simulink model "dron_filtro_complementario_version2015_RP"  (R2015b)
settings: Solver=FixedStepDiscrete  StartTime=0.0  StopTime=inf  FixedStep=0.03  RelTol=1e-3
undefined symbols (not defined in the file): DiscIntNeverNeededParam
libraries: simulink x4, arduinolib x4, RASPlib x2
settings Model: SimulationMode=external  ExtModeTrigDuration=2  Creator=jorge  LastModifiedBy=jorge
settings OptimizationCC: OptimizeModelRefInitCode=on  LifeSpan=Inf  MaxStackSize=64
settings HardwareCC: ProdBitPerInt=16  ProdBitPerPointer=16  ProdLargestAtomicFloat=None  ProdWordSize=8  ProdHWDeviceType=Atmel->AVR
settings RTWCC: SystemTargetFile=ert.tlc  TemplateMakefile=ert_default_tmf  Description=Embedded Coder  Toolchain=Arduino AVR v1.6.1  BuildConfiguration=Faster Runs
settings CodeAppCC: IgnoreCustomStorageClasses=off
settings ERTTargetCC: SupportContinuousTime=on  SupportVariableSizeSignals=on  ExtMode=on  ExtModeMexFile=ext_serial_win32_comm_rtt  ExtModeMexArgs=0 5 115200

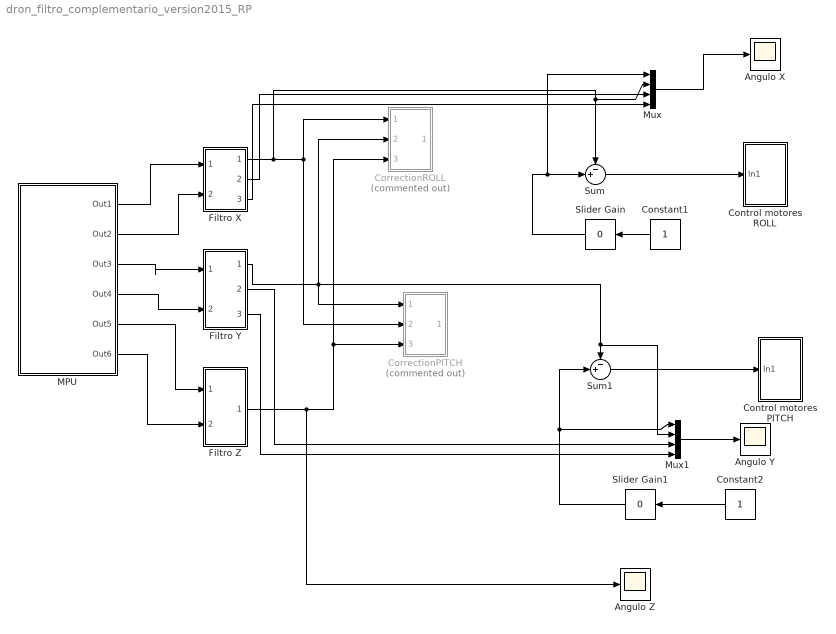
== system dron_filtro_complementario_version2015_RP ==
  Angulo X : Scope
  Angulo Y : Scope
  "Angulo Z " : Scope
  Constant1 : Constant
  Constant2 : Constant
  Control motores PITCH : Subsystem
  Control motores ROLL : Subsystem
  CorrectionPITCH : Subsystem  Commented=on
  CorrectionROLL : Subsystem  Commented=on
  Filtro X : Subsystem
  Filtro Y : Subsystem
  "Filtro Z " : Subsystem
  "MPU " : Subsystem
  Mux : Mux
  Mux1 : Mux
  Slider Gain : simulink/Math Operations/Slider Gain  low=-25  gain=0  high=35
  Slider Gain1 : simulink/Math Operations/Slider Gain  low=-25  gain=0  high=35
  Sum : Sum  Inputs=-+|
  Sum1 : Sum  Inputs=-+|
  wires:
  "MPU "/1(Out1) -> Filtro X/1(In1)
  "MPU "/2(Out2) -> Filtro X/2(In2)
  Mux/1 -> Angulo X/1
  Constant1/1 -> Slider Gain/1
  Slider Gain/1 -> Mux/1, Sum/2
  "MPU "/3(Out3) -> Filtro Y/1(In1)
  "MPU "/4(Out4) -> Filtro Y/2(In2)
  Sum/1 -> Control motores ROLL/1(In1)
  Constant2/1 -> Slider Gain1/1
  Sum1/1 -> Control motores PITCH/1(In1)
  Mux1/1 -> Angulo Y/1
  "MPU "/5(Out5) -> "Filtro Z "/1(In1)
  "MPU "/6(Out6) -> "Filtro Z "/2(In2)
  Filtro X/1(Out3) -> CorrectionPITCH/2(In2), CorrectionROLL/1(In1), Sum/1, Mux/2
  Filtro Y/1(Out3) -> CorrectionROLL/2(In2), Mux1/2, Sum1/1, CorrectionPITCH/1(In1)
  Slider Gain1/1 -> Mux1/1, Sum1/2
  "Filtro Z "/1(Out3) -> "Angulo Z "/1, CorrectionPITCH/3(In3), CorrectionROLL/3(In3)
  Filtro Y/2(Out1) -> Mux1/3
  Filtro Y/3(Out2) -> Mux1/4
  Filtro X/2(Out1) -> Mux/3
  Filtro X/3(Out2) -> Mux/4

== system dron_filtro_complementario_version2015_RP/Control motores PITCH ==
  In1 : Inport
  Control : Subsystem
  Motor1 : Subsystem
  Motor2 : Subsystem
  wires:
  In1/1 -> Control/1(In1)
  Control/1(Out1) -> Motor2/1(In1), Motor1/1(In1)

== system dron_filtro_complementario_version2015_RP/Control motores ROLL ==
  In1 : Inport
  Control : Subsystem
  Motor1 : Subsystem
  Motor2 : Subsystem
  wires:
  In1/1 -> Control/1(In1)
  Control/1(Out1) -> Motor2/1(In1), Motor1/1(In1)

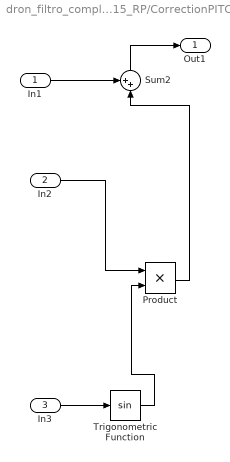
== system dron_filtro_complementario_version2015_RP/CorrectionPITCH ==
  In1 : Inport
  In2 : Inport  Port=2
  In3 : Inport  Port=3
  Product : Product
  Sum2 : Sum  Inputs=++|
  Trigonometric Function : Trigonometry
  Out1 : Outport
  wires:
  Trigonometric Function/1 -> Product/2
  Product/1 -> Sum2/2
  In1/1 -> Sum2/1
  In3/1 -> Trigonometric Function/1
  Sum2/1 -> Out1/1
  In2/1 -> Product/1

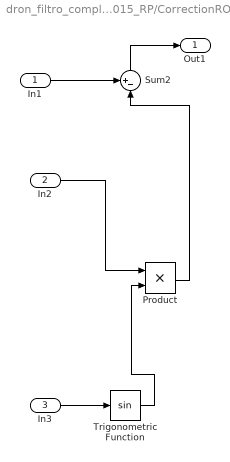
== system dron_filtro_complementario_version2015_RP/CorrectionROLL ==
  In1 : Inport
  In2 : Inport  Port=2
  In3 : Inport  Port=3
  Product : Product
  Sum2 : Sum  Inputs=+-|
  Trigonometric Function : Trigonometry
  Out1 : Outport
  wires:
  Trigonometric Function/1 -> Product/2
  Product/1 -> Sum2/2
  In1/1 -> Sum2/1
  In3/1 -> Trigonometric Function/1
  Sum2/1 -> Out1/1
  In2/1 -> Product/1

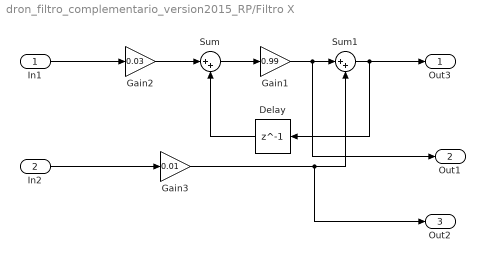
== system dron_filtro_complementario_version2015_RP/Filtro X ==
  In1 : Inport
  In2 : Inport  Port=2
  Delay : Delay  DelayLength=1  InitialCondition=0
  Gain1 : Gain  Gain=0.99
  Gain2 : Gain  Gain=0.03
  Gain3 : Gain  Gain=0.01
  Sum : Sum  Inputs=|++
  Sum1 : Sum  Inputs=|++
  Out3 : Outport
  Out1 : Outport  Port=2
  Out2 : Outport  Port=3
  wires:
  Delay/1 -> Sum/2
  Sum/1 -> Gain1/1
  In2/1 -> Gain3/1
  Gain1/1 -> Out1/1, Sum1/1
  Sum1/1 -> Out3/1, Delay/1
  In1/1 -> Gain2/1
  Gain2/1 -> Sum/1
  Gain3/1 -> Out2/1, Sum1/2

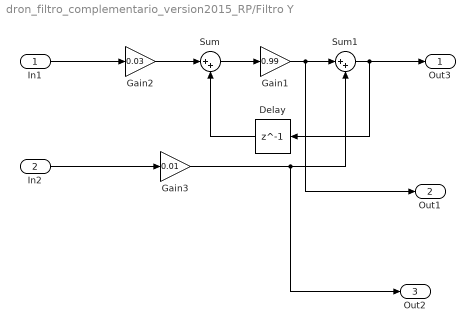
== system dron_filtro_complementario_version2015_RP/Filtro Y ==
  In1 : Inport
  In2 : Inport  Port=2
  Delay : Delay  DelayLength=1  InitialCondition=0
  Gain1 : Gain  Gain=0.99
  Gain2 : Gain  Gain=0.03
  Gain3 : Gain  Gain=0.01
  Sum : Sum  Inputs=|++
  Sum1 : Sum  Inputs=|++
  Out3 : Outport
  Out1 : Outport  Port=2
  Out2 : Outport  Port=3
  wires:
  Delay/1 -> Sum/2
  Sum/1 -> Gain1/1
  In2/1 -> Gain3/1
  Gain1/1 -> Out1/1, Sum1/1
  Sum1/1 -> Out3/1, Delay/1
  In1/1 -> Gain2/1
  Gain2/1 -> Sum/1
  Gain3/1 -> Out2/1, Sum1/2

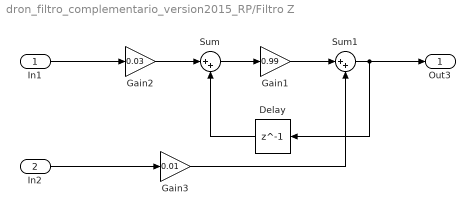
== system dron_filtro_complementario_version2015_RP/Filtro Z  ==
  In1 : Inport
  In2 : Inport  Port=2
  Delay : Delay  DelayLength=1  InitialCondition=0
  Gain1 : Gain  Gain=0.99
  Gain2 : Gain  Gain=0.03
  Gain3 : Gain  Gain=0.01
  Sum : Sum  Inputs=|++
  Sum1 : Sum  Inputs=|++
  Out3 : Outport
  wires:
  Delay/1 -> Sum/2
  Sum/1 -> Gain1/1
  In2/1 -> Gain3/1
  Gain1/1 -> Sum1/1
  Sum1/1 -> Out3/1, Delay/1
  In1/1 -> Gain2/1
  Gain2/1 -> Sum/1
  Gain3/1 -> Sum1/2

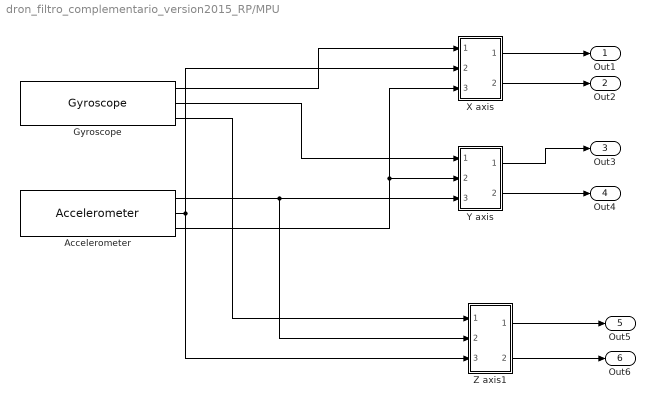
== system dron_filtro_complementario_version2015_RP/MPU  ==
  Accelerometer : RASPlib/Accelerometer  SimulateUsing=Code generation
  Gyroscope : RASPlib/Gyroscope  DLPFmode=0
  X axis : Subsystem
  Y axis : Subsystem
  Z axis1 : Subsystem
  Out1 : Outport
  Out2 : Outport  Port=2
  Out3 : Outport  Port=3
  Out4 : Outport  Port=4
  Out5 : Outport  Port=5
  Out6 : Outport  Port=6
  wires:
  Gyroscope/3 -> Z axis1/1(In1)
  Gyroscope/1 -> X axis/1(In1)
  Accelerometer/2 -> Z axis1/3(In3), X axis/2(In2)
  Accelerometer/3 -> Y axis/2(In2), X axis/3(In3)
  X axis/1(Out1) -> Out1/1
  X axis/2(Out2) -> Out2/1
  Gyroscope/2 -> Y axis/1(In1)
  Accelerometer/1 -> Y axis/3(In3), Z axis1/2(In2)
  Y axis/1(Out1) -> Out3/1
  Y axis/2(Out2) -> Out4/1
  Z axis1/2(Out2) -> Out6/1
  Z axis1/1(Out1) -> Out5/1

== system dron_filtro_complementario_version2015_RP/Control motores PITCH/Control ==
  In1 : Inport
  Clock1 : Clock
  Constant2 : Constant  Value=0
  Discrete PID Controller : simulink/Continuous/PID Controller  Controller=PID  TimeDomain=Discrete-time  SampleTime=-1  IntegratorMethod=Forward Euler  FilterMethod=Forward Euler  Form=Parallel  UseFilter=on  ControllerParametersSource=internal  P=0.11  I=0.0825  D=0.016  N=30  InitialConditionSource=internal  InitialConditionForIntegrator=0  InitialConditionForFilter=0  ExternalReset=none  LimitOutput=off  UpperSaturationLimit=inf  LowerSaturationLimit=-inf  LinearizeAsGain=off  AntiWindupMode=none  Kb=1  TrackingMode=off  Kt=1  PParamMin=[]  PParamMax=[]  IParamMin=[]  IParamMax=[]  DParamMin=[]  DParamMax=[]  NParamMin=[]  NParamMax=[]  KbParamMin=[]  KbParamMax=[]  KtParamMin=[]  KtParamMax=[]  POutMin=[]  POutMax=[]  IOutMin=[]  IOutMax=[]  DOutMin=[]  DOutMax=[]  NOutMin=[]  NOutMax=[]  KbOutMin=[]  KbOutMax=[]  KtOutMin=[]  KtOutMax=[]  IntegratorOutMin=[]  IntegratorOutMax=[]  FilterOutMin=[]  FilterOutMax=[]  SumOutMin=[]  SumOutMax=[]  SumI1OutMin=[]  SumI1OutMax=[]  SumI2OutMin=[]  SumI2OutMax=[]  SumI3OutMin=[]  SumI3OutMax=[]  SumDOutMin=[]  SumDOutMax=[]  SaturationOutMin=[]  SaturationOutMax=[]  IntegratorContinuousStateAttributes=''  IntegratorStateMustResolveToSignalObject=off  IntegratorRTWStateStorageClass=Auto  FilterContinuousStateAttributes=''  FilterStateMustResolveToSignalObject=off  FilterRTWStateStorageClass=Auto  DifferentiatorICPrevScaledInput=0  DifferentiatorOutMin=[]  DifferentiatorOutMax=[]
  Switch1 : Switch  Criteria=u2 > Threshold  Threshold=3
  Out1 : Outport
  wires:
  Discrete PID Controller/1 -> Out1/1
  Switch1/1 -> Discrete PID Controller/1
  Clock1/1 -> Switch1/2
  Constant2/1 -> Switch1/3
  In1/1 -> Switch1/1

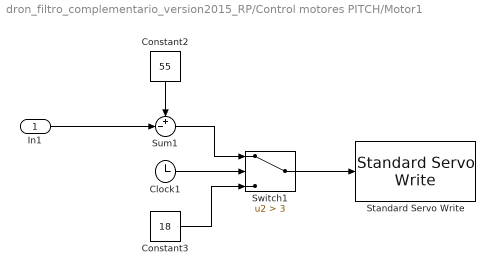
== system dron_filtro_complementario_version2015_RP/Control motores PITCH/Motor1 ==
  In1 : Inport
  Clock1 : Clock
  Constant2 : Constant  Value=55
  Constant3 : Constant  Value=18
  Standard Servo Write : arduinolib/Standard Servo Write  pinNumber=4  blockPlatform=arduino
  Sum1 : Sum  Inputs=+-|
  Switch1 : Switch  Criteria=u2 > Threshold  Threshold=3
  wires:
  In1/1 -> Sum1/2
  Constant2/1 -> Sum1/1
  Constant3/1 -> Switch1/3
  Clock1/1 -> Switch1/2
  Sum1/1 -> Switch1/1
  Switch1/1 -> Standard Servo Write/1

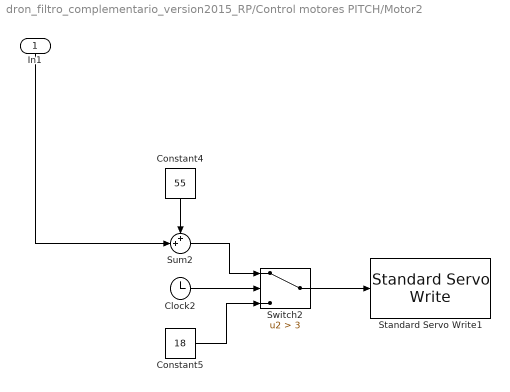
== system dron_filtro_complementario_version2015_RP/Control motores PITCH/Motor2 ==
  In1 : Inport
  Clock2 : Clock
  Constant4 : Constant  Value=55
  Constant5 : Constant  Value=18
  Standard Servo Write1 : arduinolib/Standard Servo Write  pinNumber=5  blockPlatform=arduino
  Sum2 : Sum  Inputs=++|
  Switch2 : Switch  Criteria=u2 > Threshold  Threshold=3
  wires:
  In1/1 -> Sum2/2
  Constant5/1 -> Switch2/3
  Constant4/1 -> Sum2/1
  Switch2/1 -> Standard Servo Write1/1
  Sum2/1 -> Switch2/1
  Clock2/1 -> Switch2/2

== system dron_filtro_complementario_version2015_RP/Control motores ROLL/Control ==
  In1 : Inport
  Clock1 : Clock
  Constant2 : Constant  Value=0
  Discrete PID Controller : simulink/Continuous/PID Controller  Controller=PID  TimeDomain=Discrete-time  SampleTime=-1  IntegratorMethod=Forward Euler  FilterMethod=Forward Euler  Form=Parallel  UseFilter=on  ControllerParametersSource=internal  P=0.11  I=0.0825  D=0.016  N=30  InitialConditionSource=internal  InitialConditionForIntegrator=0  InitialConditionForFilter=0  ExternalReset=none  LimitOutput=off  UpperSaturationLimit=inf  LowerSaturationLimit=-inf  LinearizeAsGain=off  AntiWindupMode=none  Kb=1  TrackingMode=off  Kt=1  PParamMin=[]  PParamMax=[]  IParamMin=[]  IParamMax=[]  DParamMin=[]  DParamMax=[]  NParamMin=[]  NParamMax=[]  KbParamMin=[]  KbParamMax=[]  KtParamMin=[]  KtParamMax=[]  POutMin=[]  POutMax=[]  IOutMin=[]  IOutMax=[]  DOutMin=[]  DOutMax=[]  NOutMin=[]  NOutMax=[]  KbOutMin=[]  KbOutMax=[]  KtOutMin=[]  KtOutMax=[]  IntegratorOutMin=[]  IntegratorOutMax=[]  FilterOutMin=[]  FilterOutMax=[]  SumOutMin=[]  SumOutMax=[]  SumI1OutMin=[]  SumI1OutMax=[]  SumI2OutMin=[]  SumI2OutMax=[]  SumI3OutMin=[]  SumI3OutMax=[]  SumDOutMin=[]  SumDOutMax=[]  SaturationOutMin=[]  SaturationOutMax=[]  IntegratorContinuousStateAttributes=''  IntegratorStateMustResolveToSignalObject=off  IntegratorRTWStateStorageClass=Auto  FilterContinuousStateAttributes=''  FilterStateMustResolveToSignalObject=off  FilterRTWStateStorageClass=Auto  DifferentiatorICPrevScaledInput=0  DifferentiatorOutMin=[]  DifferentiatorOutMax=[]
  Switch1 : Switch  Criteria=u2 > Threshold  Threshold=3
  Out1 : Outport
  wires:
  Discrete PID Controller/1 -> Out1/1
  Switch1/1 -> Discrete PID Controller/1
  Clock1/1 -> Switch1/2
  Constant2/1 -> Switch1/3
  In1/1 -> Switch1/1

== system dron_filtro_complementario_version2015_RP/Control motores ROLL/Motor1 ==
  In1 : Inport
  Clock1 : Clock
  Constant2 : Constant  Value=55
  Constant3 : Constant  Value=18
  Standard Servo Write : arduinolib/Standard Servo Write  pinNumber=2  blockPlatform=arduino
  Sum1 : Sum  Inputs=+-|
  Switch1 : Switch  Criteria=u2 > Threshold  Threshold=3
  wires:
  In1/1 -> Sum1/2
  Constant2/1 -> Sum1/1
  Constant3/1 -> Switch1/3
  Clock1/1 -> Switch1/2
  Sum1/1 -> Switch1/1
  Switch1/1 -> Standard Servo Write/1

== system dron_filtro_complementario_version2015_RP/Control motores ROLL/Motor2 ==
  In1 : Inport
  Clock2 : Clock
  Constant4 : Constant  Value=55
  Constant5 : Constant  Value=18
  Standard Servo Write1 : arduinolib/Standard Servo Write  pinNumber=3  blockPlatform=arduino
  Sum2 : Sum  Inputs=++|
  Switch2 : Switch  Criteria=u2 > Threshold  Threshold=3
  wires:
  In1/1 -> Sum2/2
  Constant5/1 -> Switch2/3
  Constant4/1 -> Sum2/1
  Switch2/1 -> Standard Servo Write1/1
  Sum2/1 -> Switch2/1
  Clock2/1 -> Switch2/2

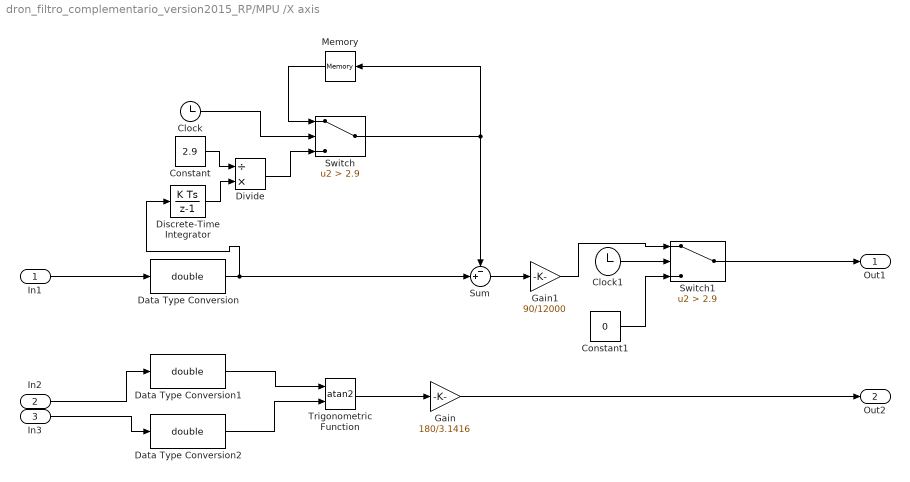
== system dron_filtro_complementario_version2015_RP/MPU /X axis ==
  In1 : Inport
  In2 : Inport  Port=2
  In3 : Inport  Port=3
  Clock : Clock
  Clock1 : Clock
  Constant : Constant  Value=2.9
  Constant1 : Constant  Value=0
  Data Type Conversion : DataTypeConversion  OutDataTypeStr=double
  Data Type Conversion1 : DataTypeConversion  OutDataTypeStr=double
  Data Type Conversion2 : DataTypeConversion  OutDataTypeStr=double
  Discrete-Time Integrator : DiscreteIntegrator  InitialConditionSetting=State (most efficient)  SampleTime=-1  ICPrevOutput=DiscIntNeverNeededParam  ICPrevScaledInput=DiscIntNeverNeededParam
  Divide : Product  Inputs=/*
  Gain : Gain  Gain=180/3.1416
  Gain1 : Gain  Gain=90/12000
  Memory : Memory
  Sum : Sum  Inputs=-+|
  Switch : Switch  Criteria=u2 > Threshold  Threshold=2.9
  Switch1 : Switch  Criteria=u2 > Threshold  Threshold=2.9
  Trigonometric Function : Trigonometry  Operator=atan2
  Out1 : Outport
  Out2 : Outport  Port=2
  wires:
  Sum/1 -> Gain1/1
  Clock/1 -> Switch/2
  Switch/1 -> Sum/1, Memory/1
  Constant/1 -> Divide/1
  Gain/1 -> Out2/1
  Clock1/1 -> Switch1/2
  Trigonometric Function/1 -> Gain/1
  Data Type Conversion/1 -> Sum/2, Discrete-Time Integrator/1
  Switch1/1 -> Out1/1
  Data Type Conversion1/1 -> Trigonometric Function/1
  Data Type Conversion2/1 -> Trigonometric Function/2
  In2/1 -> Data Type Conversion1/1
  Constant1/1 -> Switch1/3
  In3/1 -> Data Type Conversion2/1
  Divide/1 -> Switch/3
  Memory/1 -> Switch/1
  Discrete-Time Integrator/1 -> Divide/2
  In1/1 -> Data Type Conversion/1
  Gain1/1 -> Switch1/1

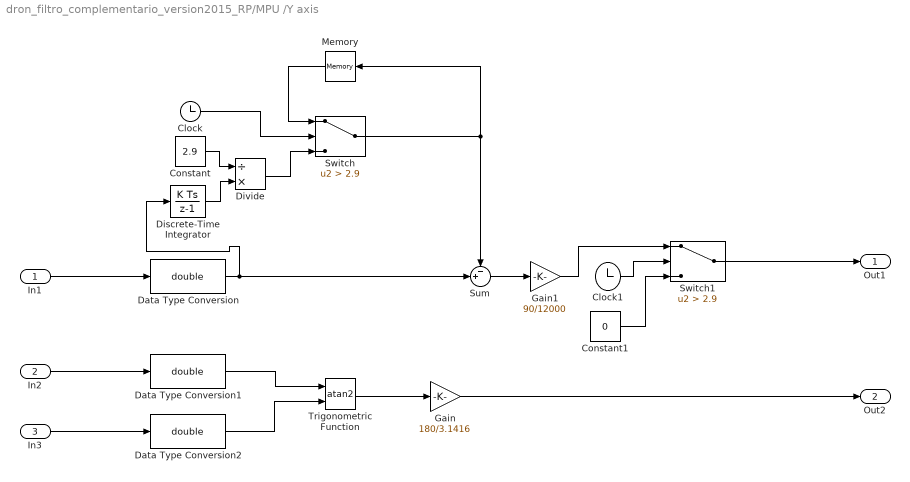
== system dron_filtro_complementario_version2015_RP/MPU /Y axis ==
  In1 : Inport
  In2 : Inport  Port=2
  In3 : Inport  Port=3
  Clock : Clock
  Clock1 : Clock
  Constant : Constant  Value=2.9
  Constant1 : Constant  Value=0
  Data Type Conversion : DataTypeConversion  OutDataTypeStr=double
  Data Type Conversion1 : DataTypeConversion  OutDataTypeStr=double
  Data Type Conversion2 : DataTypeConversion  OutDataTypeStr=double
  Discrete-Time Integrator : DiscreteIntegrator  InitialConditionSetting=State (most efficient)  SampleTime=-1  ICPrevOutput=DiscIntNeverNeededParam  ICPrevScaledInput=DiscIntNeverNeededParam
  Divide : Product  Inputs=/*
  Gain : Gain  Gain=180/3.1416
  Gain1 : Gain  Gain=90/12000
  Memory : Memory
  Sum : Sum  Inputs=-+|
  Switch : Switch  Criteria=u2 > Threshold  Threshold=2.9
  Switch1 : Switch  Criteria=u2 > Threshold  Threshold=2.9
  Trigonometric Function : Trigonometry  Operator=atan2
  Out1 : Outport
  Out2 : Outport  Port=2
  wires:
  Sum/1 -> Gain1/1
  Clock/1 -> Switch/2
  Switch/1 -> Sum/1, Memory/1
  Constant/1 -> Divide/1
  Gain/1 -> Out2/1
  Clock1/1 -> Switch1/2
  Trigonometric Function/1 -> Gain/1
  Data Type Conversion/1 -> Sum/2, Discrete-Time Integrator/1
  Switch1/1 -> Out1/1
  Data Type Conversion1/1 -> Trigonometric Function/1
  Data Type Conversion2/1 -> Trigonometric Function/2
  In2/1 -> Data Type Conversion1/1
  Constant1/1 -> Switch1/3
  In3/1 -> Data Type Conversion2/1
  Divide/1 -> Switch/3
  Memory/1 -> Switch/1
  Discrete-Time Integrator/1 -> Divide/2
  In1/1 -> Data Type Conversion/1
  Gain1/1 -> Switch1/1

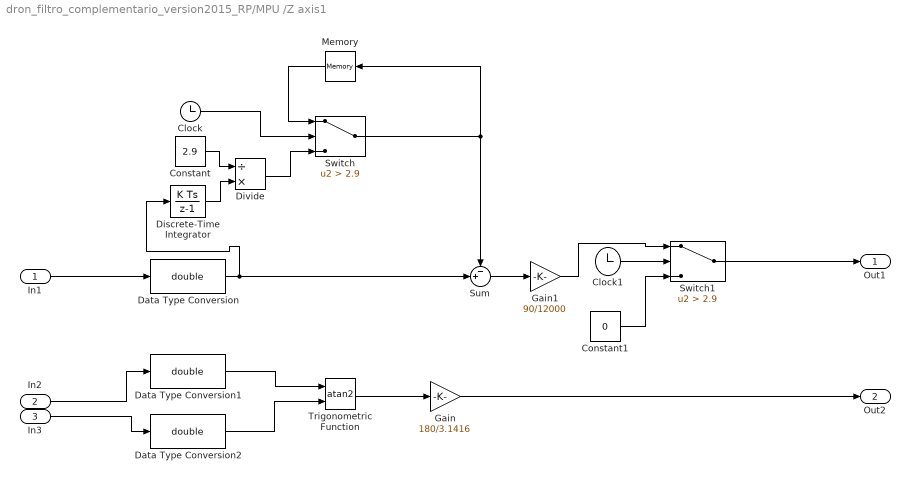
== system dron_filtro_complementario_version2015_RP/MPU /Z axis1 ==
  In1 : Inport
  In2 : Inport  Port=2
  In3 : Inport  Port=3
  Clock : Clock
  Clock1 : Clock
  Constant : Constant  Value=2.9
  Constant1 : Constant  Value=0
  Data Type Conversion : DataTypeConversion  OutDataTypeStr=double
  Data Type Conversion1 : DataTypeConversion  OutDataTypeStr=double
  Data Type Conversion2 : DataTypeConversion  OutDataTypeStr=double
  Discrete-Time Integrator : DiscreteIntegrator  InitialConditionSetting=State (most efficient)  SampleTime=-1  ICPrevOutput=DiscIntNeverNeededParam  ICPrevScaledInput=DiscIntNeverNeededParam
  Divide : Product  Inputs=/*
  Gain : Gain  Gain=180/3.1416
  Gain1 : Gain  Gain=90/12000
  Memory : Memory
  Sum : Sum  Inputs=-+|
  Switch : Switch  Criteria=u2 > Threshold  Threshold=2.9
  Switch1 : Switch  Criteria=u2 > Threshold  Threshold=2.9
  Trigonometric Function : Trigonometry  Operator=atan2
  Out1 : Outport
  Out2 : Outport  Port=2
  wires:
  Sum/1 -> Gain1/1
  Clock/1 -> Switch/2
  Switch/1 -> Sum/1, Memory/1
  Constant/1 -> Divide/1
  Gain/1 -> Out2/1
  Clock1/1 -> Switch1/2
  Trigonometric Function/1 -> Gain/1
  Data Type Conversion/1 -> Sum/2, Discrete-Time Integrator/1
  Switch1/1 -> Out1/1
  Data Type Conversion1/1 -> Trigonometric Function/1
  Data Type Conversion2/1 -> Trigonometric Function/2
  In2/1 -> Data Type Conversion1/1
  Constant1/1 -> Switch1/3
  In3/1 -> Data Type Conversion2/1
  Divide/1 -> Switch/3
  Memory/1 -> Switch/1
  Discrete-Time Integrator/1 -> Divide/2
  In1/1 -> Data Type Conversion/1
  Gain1/1 -> Switch1/1
